simulink model "filtration1210"  (R2024a)
settings: Solver=VariableStepAuto  StartTime=0.0  StopTime=20770.8  MaxStep=0.1  RelTol=1e-3
undefined symbols (not defined in the file): fdesignblkfcn, gcbh
libraries: dspstat3 x1, dsparch4 x1
settings Model: Creator=pupkinzalupkin  LastModifiedBy=pupkinzalupkin

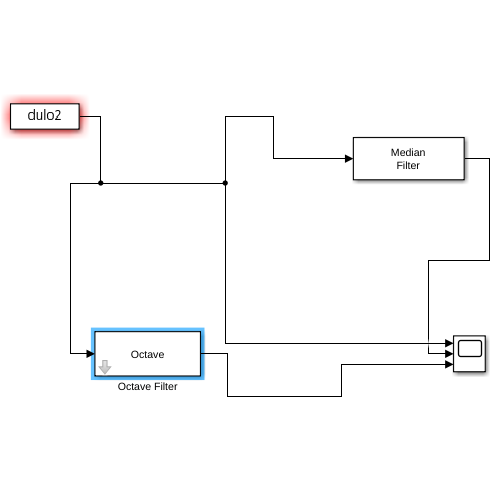
[thumbnail: Simulink's stored preview of the top-level diagram]
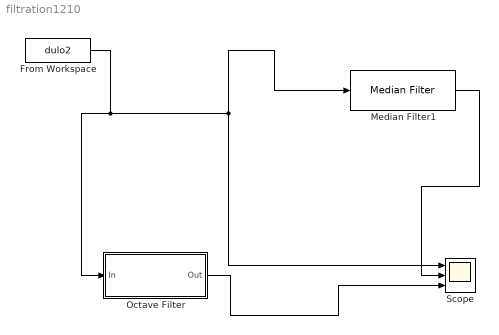
== system filtration1210 ==
  From Workspace : FromWorkspace  VariableName=dulo2
  Median Filter1 : dspstat3/Median Filter  WindowLength=100  SimulateUsing=Interpreted execution
      settings: LibrarySourceBlock=|
      | dspfdesign/Median
      | Filter
  Octave Filter : Subsystem  DialogController=fdesignblkfcn  InitFcn=fdesignblkfcn(gcbh, {'InitFcn'});  mask(Octave Filter){}
      mask help: dsp:DSPFilterDesignBlockDialog:OctaveFdesign_MaskDesc
      settings: CopyFcn=fdesignblkfcn(gcbh, {'CopyFcn'});
      mask Help: helpview(mapfilelocation('dsp'), 'dspoctavefilter');
      mask Display: disp('Octave');
  Scope : Scope  NumInputPorts=3
  wires:
  From Workspace/1 -> Scope/1, Median Filter1/1, Octave Filter/1(In)
  Median Filter1/1 -> Scope/2
  Octave Filter/1(Out) -> Scope/3

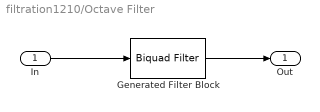
== system filtration1210/Octave Filter ==
  In : Inport
  Generated Filter Block : dsparch4/Biquad Filter  Tag=BlockMethodSubSystem  FilterSource=Dialog parameters  CoeffSource=Specify via dialog  FilterObject=BQF  IIRFiltStruct=Direct form II  BiQuadCoeffs=[0.00504841112148836976 0 -0.00504841112148836976 1 -1.99992284077516569 0.999922842426619107;0.000137958644296090339 0 -0.000137958644296090339 1 -1.99989298114073066 0.999893141529221374;2 0 -2 1 -1.99981592399091546 0.99981599219922701]  ScaleValues=[1.65145341846084648e-09;1;1;338.5779845735251]  IC=0  ICnum=0  ICden=0  a0Flag=Warning  optimizeScaleValues=off  ScaleValueMode=Specify via input port (g)  InputProcessing=Columns as channels (frame based)  roundingMode=Floor  overflowMode=off  scaleValueFracLength=14  denProdOutputFracLength=30  denAccumFracLength=30  secondMemoryFracLength=15
  Out : Outport  VectorParamsAs1DForOutWhenUnconnected=off
  wires:
  Generated Filter Block/1 -> Out/1
  In/1 -> Generated Filter Block/1
